simulink model "Kalman_Filter_with_LQR"  (R2021a)
settings: Solver=VariableStepAuto  StartTime=0.0  StopTime=10.0  RelTol=1e-3
values from neighbouring files (symbols this model uses):
  A = [0 1 0 0 ... (first row only)    [Controllability_of_a_Linear_System.m]    (also in Full_State_Feedback_Control_Design.m = [0 3;2 4]; Implementation_Issues_with_a_FSFB.m = [0 1 0; Introduction_to_Full_State_Feedback_COntrol.m = [0 3;2 4]; Introduction_to_LQR_control.m = [0 1)
  B = [0 ... (first row only)    [Controllability_of_a_Linear_System.m]    (also in Full_State_Feedback_Control_Design.m = [-2 1; 1 1]; Implementation_Issues_with_a_FSFB.m = [0 0; Introduction_to_Full_State_Feedback_COntrol.m = [-2 1; 1 1]; Introduction_to_LQR_control.m)
  C = eye(3)    [Implementation_Issues_with_a_FSFB.m]    (also in Kalman_Filter_Design.m = [1 0 0 0]; Observability_example.m = [1 0 0 1]; Observability_gramion_example.m = [0 0 1]; Practical_Implementation_Issues_with_a_FSFB.m)
  K = place(A,B(:,1),desired_closed_loop_poles)    [Implementation_Issues_with_a_FSFB.m]    (also in Practical_Implementation_Issues_with_a_FSFB.m)
  Vn = 1    [Kalman_Filter_Design.m]
  x0 = [72*pi/180 ... (first row only)    [Implementation_Issues_with_a_FSFB.m]    (also in Introduction_to_LQR_control.m = [pi; Kalman_Filter_Design.m = [0;-2;-pi/2;2]; LQR_control.m = [pi)
undefined symbols (not defined in the file or in its folder): Continuous, Time
libraries: ctrlSharedLib x2, simulink x1
settings Model: Creator=subhi  LastModifiedBy=subhi

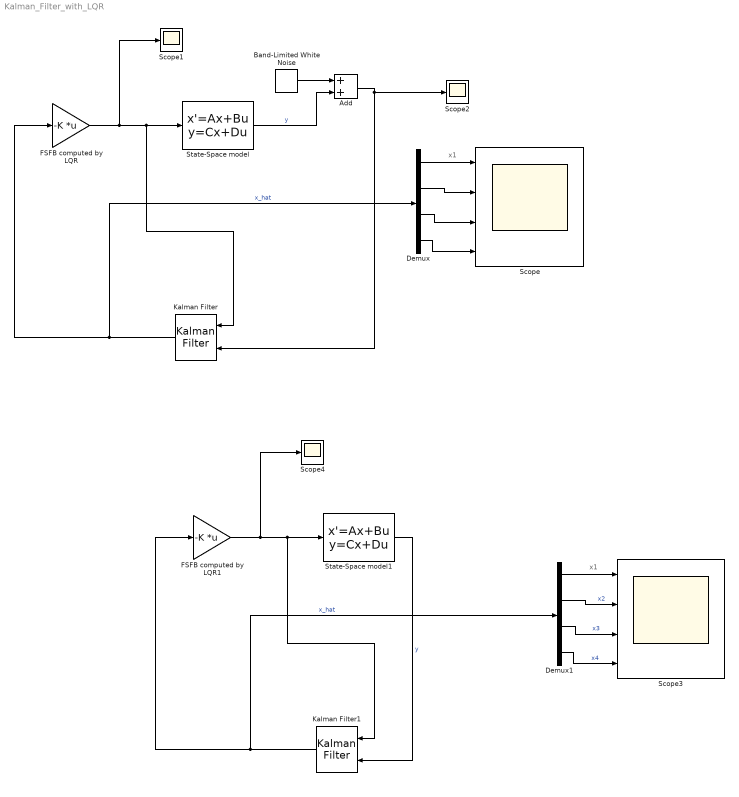
== system Kalman_Filter_with_LQR ==
  note: x1
  note: x1
  Add : Sum
  Band-Limited White Noise : simulink/Sources/Band-Limited White Noise  Cov=[0.1]  Ts=0.1  seed=[23341]
  Demux : Demux
  Demux1 : Demux
  FSFB computed by LQR : Gain  Gain=-K  Multiplication=Matrix(K*u)
  FSFB computed by LQR1 : Gain  Gain=-K  Multiplication=Matrix(K*u)
  Kalman Filter : ctrlSharedLib/Kalman Filter  TimeDomain=Continuous-Time  UseCurrentEstimator=on  ModelSource=Individual A, B, C, D matrices  ModelSourceVariable=ss(0.95,1,1,0,1)  A=A  B=B  C=C  D=zeros(size(C,1),size(B,2))  NumberOfStates=1  NumberOfInputs=1  NumberOfOutputs=1  InitialEstimateSource=Dialog  X0=0  P0=10  UseK=off  UseGH=off  NumberOfProcessNoiseInputs=1  G=1  TimeInvariantG=on  H=0  TimeInvariantH=on  Q=Vd  TimeInvariantQ=on  R=Vn  TimeInvariantR=on  N=0  TimeInvariantN=on  AddInputPort=on  AddEnablePort=off  OutputEstimatedY=off  OutputP=off  Ts=-1
  Kalman Filter1 : ctrlSharedLib/Kalman Filter  TimeDomain=Continuous-Time  UseCurrentEstimator=on  ModelSource=Individual A, B, C, D matrices  ModelSourceVariable=ss(0.95,1,1,0,1)  A=A  B=B  C=C  D=zeros(size(C,1),size(B,2))  NumberOfStates=1  NumberOfInputs=1  NumberOfOutputs=1  InitialEstimateSource=Dialog  X0=0  P0=10  UseK=off  UseGH=off  NumberOfProcessNoiseInputs=1  G=1  TimeInvariantG=on  H=0  TimeInvariantH=on  Q=Vd  TimeInvariantQ=on  R=Vn  TimeInvariantR=on  N=0  TimeInvariantN=on  AddInputPort=on  AddEnablePort=off  OutputEstimatedY=off  OutputP=off  Ts=-1
  Scope : Scope  NumInputPorts=4
  Scope1 : Scope
  Scope2 : Scope
  Scope3 : Scope  NumInputPorts=4
  Scope4 : Scope
  State-Space model : StateSpace  A=A  B=B  C=C  D=zeros(size(C,1),size(B,2))  InitialCondition=x0
  State-Space model1 : StateSpace  A=A  B=B  C=C  D=zeros(size(C,1),size(B,2))  InitialCondition=x0
  wires:
  FSFB computed by LQR/1 -> Kalman Filter/1, State-Space model/1, Scope1/1
  Demux/1 -> Scope/1
  State-Space model/1 -> Add/2  "y"
  Kalman Filter/1 -> Demux/1, FSFB computed by LQR/1  "x_hat"
  Demux/2 -> Scope/2
  Demux/3 -> Scope/3
  Demux/4 -> Scope/4
  Band-Limited White Noise/1 -> Add/1
  Add/1 -> Kalman Filter/2, Scope2/1
  Demux1/3 -> Scope3/3  "x3"
  Demux1/4 -> Scope3/4  "x4"
  Kalman Filter1/1 -> Demux1/1, FSFB computed by LQR1/1  "x_hat"
  FSFB computed by LQR1/1 -> Kalman Filter1/1, State-Space model1/1, Scope4/1
  Demux1/2 -> Scope3/2  "x2"
  Demux1/1 -> Scope3/1
  State-Space model1/1 -> Kalman Filter1/2  "y"
